simulink model "smc_demo"  (Simulink 10.3)
settings: Solver=ode45  StartTime=0.0  StopTime=20  RelTol=1e-3  EnableMultiTasking=on
settings Model: Creator=ljk  LastModifiedBy=YuTaov5  ExtModeTrigMode=oneshot  ExtModeArmWhenConnect=off
settings DataIOCC: SignalLoggingName=sigsOut
settings OptimizationCC: BooleanDataType=off
settings DebuggingCC: SaveWithParameterizedLinksMsg=none  SignalResolutionControl=TryResolveAllWithWarning  MultiTaskDSMMsg=warning  MultiTaskCondExecSysMsg=none
settings HardwareCC: TargetUnknown=on

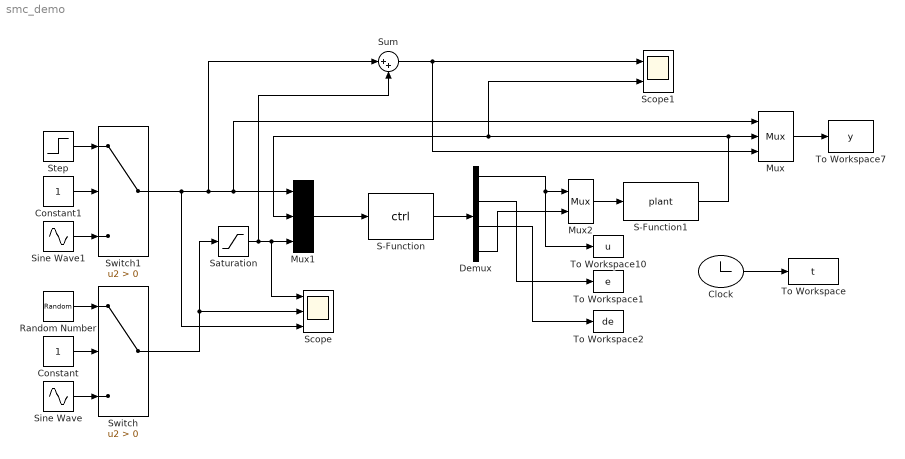
== system smc_demo ==
  Clock : Clock
  Constant : Constant
  Constant1 : Constant
  Demux : Demux
      settings: DisplayOption=none
  Mux : Mux  Inputs=3
  Mux1 : Mux  Inputs=3
  Mux2 : Mux  Inputs=2
  Random Number : RandomNumber  Variance=0.2  SampleTime=0
  S-Function : S-Function  FunctionName=ctrl  SFunctionDeploymentMode=off  EnableBusSupport=off
  S-Function1 : S-Function  FunctionName=plant  SFunctionDeploymentMode=off  EnableBusSupport=off
  Saturation : Saturate
  Scope : Scope  NumInputPorts=3
  Scope1 : Scope  NumInputPorts=2
  Sine Wave : Sin  Amplitude=0.2  Frequency=10  SampleTime=0
  Sine Wave1 : Sin  SampleTime=0
  Step : Step  Time=0  SampleTime=0
  Sum : Sum  Inputs=|++
  Switch : Switch  Criteria=u2 > Threshold
  Switch1 : Switch  Criteria=u2 > Threshold
  To Workspace : ToWorkspace  VariableName=t  SampleTime=-1
  To Workspace1 : ToWorkspace  VariableName=e  SampleTime=-1
  To Workspace10 : ToWorkspace  VariableName=u  SampleTime=-1
  To Workspace2 : ToWorkspace  VariableName=de  SampleTime=-1
  To Workspace7 : ToWorkspace  VariableName=y  SampleTime=-1
  wires:
  Switch1/1 -> Scope/3, Sum/1, Mux/1, Mux1/1
  Mux1/1 -> S-Function/1
  Clock/1 -> To Workspace/1
  Mux/1 -> To Workspace7/1
  S-Function1/1 -> Mux1/2, Scope1/2, Mux/2
  S-Function/1 -> Demux/1
  Demux/1 -> To Workspace10/1, Mux2/1
  Demux/3 -> To Workspace2/1
  Demux/2 -> To Workspace1/1
  Saturation/1 -> Scope/1, Mux1/3, Sum/2
  Demux/4 -> Mux2/2
  Mux2/1 -> S-Function1/1
  Constant/1 -> Switch/2
  Switch/1 -> Saturation/1, Scope/2
  Random Number/1 -> Switch/1
  Sine Wave/1 -> Switch/3
  Sum/1 -> Mux/3, Scope1/1
  Step/1 -> Switch1/1
  Sine Wave1/1 -> Switch1/3
  Constant1/1 -> Switch1/2
